simulink model "systema"  (R2017b)
settings: Solver=ode4  StartTime=0.0  StopTime=10  FixedStep=0.01  RelTol=1e-3  EnableMultiTasking=on
libraries: simulink x14
CloseFcn:
  | rtwprivate ssgencode ModelCloseRequest systema
settings Model: Creator=ece  LastModifiedBy=lenovo
settings DataIOCC: SaveFormat=Array  SignalLoggingName=sigsOut
settings OptimizationCC: OptimizeBlockIOStorage=off  BufferReuse=off  GlobalBufferReuse=off  ExpressionFolding=off  ExpressionDepthLimit=2147483647  LocalBlockOutputs=off  InitFltsAndDblsToZero=on  LifeSpan=inf
settings DebuggingCC: SaveWithParameterizedLinksMsg=none  UnderspecifiedInitializationDetection=Classic  MergeDetectMultiDrivingBlocksExec=none  SignalResolutionControl=TryResolveAllWithWarning  MultiTaskDSMMsg=warning  MultiTaskCondExecSysMsg=none  FcnCallInpInsideContextMsg=warning  AllowSymbolicDim=off  StateNameClashWarn=warning  SFUnexpectedBacktrackingDiag=warning  SFNoUnconditionalDefaultTransitionDiag=warning  SFExecutionAtInitializationDiag=none
settings HardwareCC: ProdBitPerPointer=32  ProdBitPerSizeT=32  ProdBitPerPtrDiffT=32  ProdLargestAtomicFloat=None  ProdIntDivRoundTo=Undefined  ProdEndianess=Unspecified  ProdWordSize=32  ProdHWDeviceType=32-bit Generic  TargetUnknown=on
settings ModelReferenceCC: PropagateSignalLabelsOutOfModel=off
settings CodeAppCC: StateflowObjectComments=on
settings GRTTargetCC: TargetFcnLib=ansi_tfl_tmw.mat  TargetLangStandard=C89/C90 (ANSI)  ModelReferenceCompliant=off  GeneratePreprocessorConditionals=Disable all  CombineOutputUpdateFcns=off  MatFileLogging=off  GRTInterface=on
settings ConfigComp: CovMetricSettings=dw  CovHtmlReporting=on  CovSaveCumulativeToWorkspaceVar=on  CovSaveSingleToWorkspaceVar=on  CovExternalEMLEnable=off

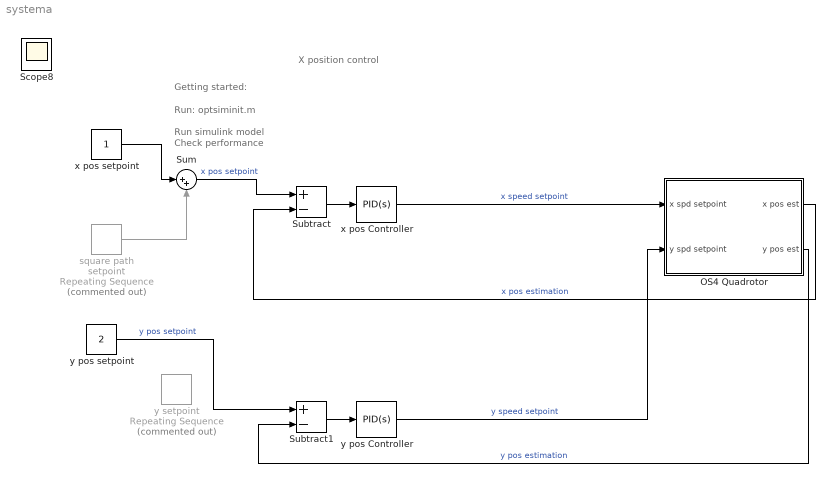
== system systema ==
  note: Check performance
  note: Run simulink model
  note: Run: optsiminit.m
  note: Getting started:
  note: X position control
  OS4 Quadrotor : Subsystem
  Subtract : Sum  Inputs=+-
  Subtract1 : Sum  Inputs=+-
  Sum : Sum  Inputs=|++
  square path setpoint : simulink/Sources/Repeating Sequence  Commented=on  rep_seq_t=[0 5 9.99 10 15 19.99 20 25]  rep_seq_y="[0 1 1       1 1 1 1 1]"
  x pos Controller : simulink/Continuous/PID Controller  Controller=PID  TimeDomain=Continuous-time  SampleTime=-1  IntegratorMethod=Forward Euler  FilterMethod=Forward Euler  Form=Parallel  UseFilter=on  ControllerParametersSource=internal  P=1.78976019221014  I=0.309124158830126  D=1.80752216558791  N=4.82597653544632  InitialConditionSource=internal  InitialConditionForIntegrator=0  InitialConditionForFilter=0  ExternalReset=none  LimitOutput=off  UpperSaturationLimit=inf  LowerSaturationLimit=-inf  LinearizeAsGain=off  AntiWindupMode=none  Kb=1  TrackingMode=off  Kt=1  PParamMin=[]  PParamMax=[]  IParamMin=[]  IParamMax=[]  DParamMin=[]  DParamMax=[]  NParamMin=[]  NParamMax=[]  KbParamMin=[]  KbParamMax=[]  KtParamMin=[]  KtParamMax=[]  POutMin=[]  POutMax=[]  IOutMin=[]  IOutMax=[]  DOutMin=[]  DOutMax=[]  NOutMin=[]  NOutMax=[]  KbOutMin=[]  KbOutMax=[]  KtOutMin=[]  KtOutMax=[]  IntegratorOutMin=[]  IntegratorOutMax=[]  FilterOutMin=[]  FilterOutMax=[]  SumOutMin=[]  SumOutMax=[]  SumI1OutMin=[]  SumI1OutMax=[]  SumI2OutMin=[]  SumI2OutMax=[]  SumI3OutMin=[]  SumI3OutMax=[]  SumDOutMin=[]  SumDOutMax=[]  SaturationOutMin=[]  SaturationOutMax=[]  IntegratorContinuousStateAttributes=''  IntegratorStateMustResolveToSignalObject=off  IntegratorRTWStateStorageClass=Auto  FilterContinuousStateAttributes=''  FilterStateMustResolveToSignalObject=off  FilterRTWStateStorageClass=Auto  DifferentiatorICPrevScaledInput=0  DifferentiatorOutMin=[]  DifferentiatorOutMax=[]  InitialConditionSetting=State (most efficient)  FilterDiffOutCoefMin=[]  FilterDiffOutCoefMax=[]  SumDenOutMin=[]  SumDenOutMax=[]  SumNumOutMin=[]  SumNumOutMax=[]  ReciprocalOutMin=[]  ReciprocalOutMax=[]  DivideOutMin=[]  DivideOutMax=[]  TunerSelectOption=Transfer Function Based (PID Tuner App)
  x pos setpoint : Constant
  y pos Controller : simulink/Continuous/PID Controller  Controller=PID  TimeDomain=Continuous-time  SampleTime=-1  IntegratorMethod=Forward Euler  FilterMethod=Forward Euler  Form=Parallel  UseFilter=on  ControllerParametersSource=internal  P=1  I=0.2  D=0  N=100  InitialConditionSource=internal  InitialConditionForIntegrator=0  InitialConditionForFilter=0  ExternalReset=none  LimitOutput=off  UpperSaturationLimit=inf  LowerSaturationLimit=-inf  LinearizeAsGain=off  AntiWindupMode=none  Kb=1  TrackingMode=off  Kt=1  PParamMin=[]  PParamMax=[]  IParamMin=[]  IParamMax=[]  DParamMin=[]  DParamMax=[]  NParamMin=[]  NParamMax=[]  KbParamMin=[]  KbParamMax=[]  KtParamMin=[]  KtParamMax=[]  POutMin=[]  POutMax=[]  IOutMin=[]  IOutMax=[]  DOutMin=[]  DOutMax=[]  NOutMin=[]  NOutMax=[]  KbOutMin=[]  KbOutMax=[]  KtOutMin=[]  KtOutMax=[]  IntegratorOutMin=[]  IntegratorOutMax=[]  FilterOutMin=[]  FilterOutMax=[]  SumOutMin=[]  SumOutMax=[]  SumI1OutMin=[]  SumI1OutMax=[]  SumI2OutMin=[]  SumI2OutMax=[]  SumI3OutMin=[]  SumI3OutMax=[]  SumDOutMin=[]  SumDOutMax=[]  SaturationOutMin=[]  SaturationOutMax=[]  IntegratorContinuousStateAttributes=''  IntegratorStateMustResolveToSignalObject=off  IntegratorRTWStateStorageClass=Auto  FilterContinuousStateAttributes=''  FilterStateMustResolveToSignalObject=off  FilterRTWStateStorageClass=Auto  DifferentiatorICPrevScaledInput=0  DifferentiatorOutMin=[]  DifferentiatorOutMax=[]  InitialConditionSetting=State (most efficient)  FilterDiffOutCoefMin=[]  FilterDiffOutCoefMax=[]  SumDenOutMin=[]  SumDenOutMax=[]  SumNumOutMin=[]  SumNumOutMax=[]  ReciprocalOutMin=[]  ReciprocalOutMax=[]  DivideOutMin=[]  DivideOutMax=[]  TunerSelectOption=Transfer Function Based (PID Tuner App)
  y pos setpoint : Constant  Value=2
  y setpoint : simulink/Sources/Repeating Sequence  Commented=on  rep_seq_t=[0 4.99 5 10 14.99 15 20 25]  rep_seq_y="[2 2   4 4 4 2 2 2]"
  Scope8 : Scope
  wires:
  Sum/1 -> Subtract/1  "x pos setpoint"
  Subtract/1 -> x pos Controller/1
  x pos Controller/1 -> OS4 Quadrotor/1(x spd setpoint)  "x speed setpoint"
  OS4 Quadrotor/1(x pos est) -> Subtract/2  "x pos estimation"
  square path setpoint/1 -> Sum/2
  x pos setpoint/1 -> Sum/1
  y pos setpoint/1 -> Subtract1/1  "y pos setpoint"
  Subtract1/1 -> y pos Controller/1
  y pos Controller/1 -> OS4 Quadrotor/2(y spd setpoint)  "y speed setpoint"
  OS4 Quadrotor/2(y pos est) -> Subtract1/2  "y pos estimation"

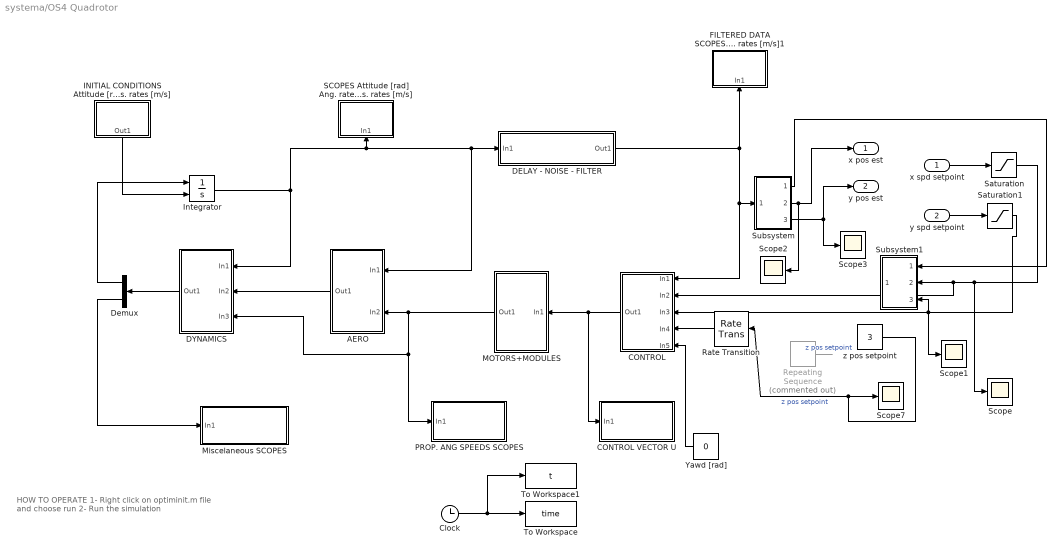
== system systema/OS4 Quadrotor ==
  note: HOW TO OPERATE
      | 1- Right click on optiminit.m file and choose run
      | 2- Run the simulation
  x spd setpoint : Inport
  y spd setpoint : Inport  Port=2
  AERO : Subsystem
  CONTROL : Subsystem
  CONTROL VECTOR U : Subsystem
  Clock : Clock
  DELAY - NOISE - FILTER : Subsystem
  DYNAMICS : Subsystem
  Demux : Demux  Outputs=2
  FILTERED DATA SCOPES Attitude [rad] Ang. rates [rad/sec] position [m] Pos. rates [m/s]1 : Subsystem
  "INITIAL CONDITIONS Attitude [rad] Ang. rates [rad/sec] position [m] Pos. rates [m/s] " : Subsystem
  Integrator : Integrator  InitialConditionSource=external
  MOTORS+MODULES : Subsystem
  Miscelaneous SCOPES : Subsystem
  PROP. ANG SPEEDS SCOPES : Subsystem
  Rate Transition : RateTransition
  Repeating Sequence : simulink/Sources/Repeating Sequence  Commented=on  rep_seq_t=[0 5 9.99 10 15 19.99 20 25]  rep_seq_y="[3 3 3       5 5 5 3 3]"
  SCOPES Attitude [rad] Ang. rates [rad/sec] position [m] Pos. rates [m/s] : Subsystem
  Saturation : Saturate  UpperLimit=20  LowerLimit=-20
  Saturation1 : Saturate  UpperLimit=20  LowerLimit=-20
  Scope{,1..3,7} (5 alike) : Scope
  Subsystem : Subsystem
  Subsystem1 : Subsystem
  To Workspace : ToWorkspace  VariableName=time  SampleTime=-1
  To Workspace1 : ToWorkspace  VariableName=t  SampleTime=-1
  Yawd [rad] : Constant  Value=0
  z pos setpoint : Constant  Value=3
  x pos est : Outport
  y pos est : Outport  Port=2
  wires:
  z pos setpoint/1 -> Scope7/1, Rate Transition/1  "z pos setpoint"
  Rate Transition/1 -> CONTROL/4(In4)
  y spd setpoint/1 -> Saturation1/1
  Saturation1/1 -> CONTROL/3(In3), Subsystem1/3(In3), Scope1/1
  Saturation/1 -> Scope/1, Subsystem1/2(In2), CONTROL/2(In2)
  x spd setpoint/1 -> Saturation/1
  Subsystem/1(Out2) -> Subsystem1/1(In1)
  Subsystem/2(Out3) -> x pos est/1, Scope2/1
  Subsystem/3(Out4) -> y pos est/1, Scope3/1
  DELAY - NOISE - FILTER/1(Out1) -> FILTERED DATA SCOPES Attitude [rad] Ang. rates [rad/sec] position [m] Pos. rates [m/s]1/1(In1), CONTROL/1(In1), Subsystem/1(In1)
  AERO/1(Out1) -> DYNAMICS/2(In2)
  MOTORS+MODULES/1(Out1) -> AERO/2(In2), DYNAMICS/3(In3), PROP. ANG SPEEDS SCOPES/1(In1)
  Yawd [rad]/1 -> CONTROL/5(In5)
  Demux/1 -> Integrator/1
  CONTROL/1(Out1) -> MOTORS+MODULES/1(In1), CONTROL VECTOR U/1(In1)
  Demux/2 -> Miscelaneous SCOPES/1(In1)
  DYNAMICS/1(Out1) -> Demux/1
  Clock/1 -> To Workspace/1, To Workspace1/1
  "INITIAL CONDITIONS Attitude [rad] Ang. rates [rad/sec] position [m] Pos. rates [m/s] "/1(Out1) -> Integrator/2
  Integrator/1 -> SCOPES Attitude [rad] Ang. rates [rad/sec] position [m] Pos. rates [m/s]/1(In1), DELAY - NOISE - FILTER/1(In1), AERO/1(In1), DYNAMICS/1(In1)
  Repeating Sequence/1 -> ?  "z pos setpoint"

== system systema/OS4 Quadrotor/AERO ==
  In1 : Inport
  In2 : Inport  Port=2
  AERO Attitude [rad] : MATLABFcn  MATLABFcn=aero  OutputDimensions=24
  Mux1 : Mux  Inputs=2
  Out1 : Outport
  wires:
  In1/1 -> Mux1/1
  In2/1 -> Mux1/2
  Mux1/1 -> AERO Attitude [rad]/1
  AERO Attitude [rad]/1 -> Out1/1

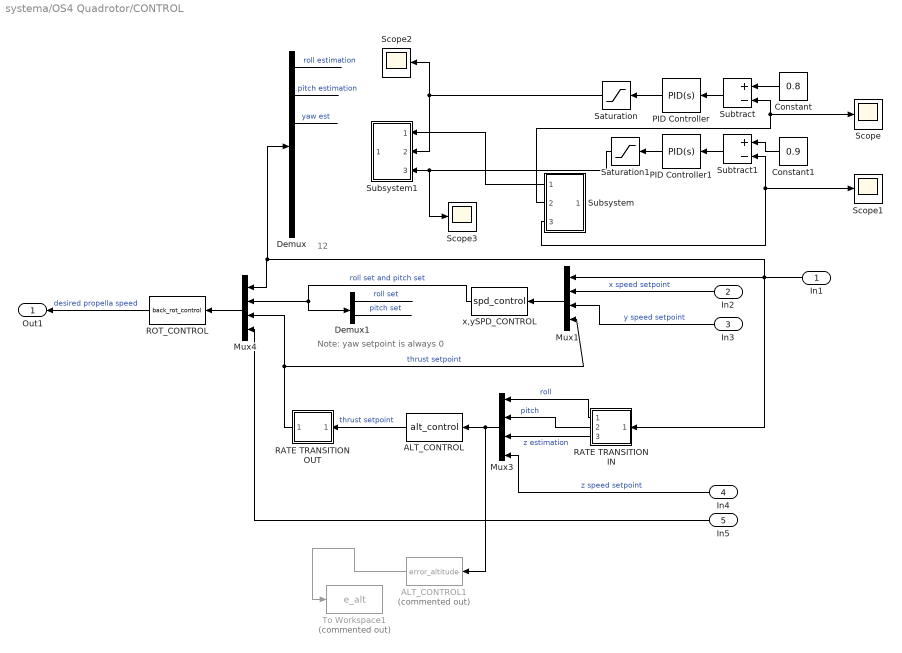
== system systema/OS4 Quadrotor/CONTROL ==
  note: Note: yaw setpoint is always 0
  note: 12
  In1 : Inport
  In2 : Inport  Port=2
  In3 : Inport  Port=3
  In4 : Inport  Port=4
  In5 : Inport  Port=5
  ALT_CONTROL : MATLABFcn  MATLABFcn=alt_control  OutputDimensions=1  SampleTime=0.05
  ALT_CONTROL1 : MATLABFcn  Commented=on  MATLABFcn=error_altitude  OutputDimensions=1  SampleTime=0.05
  Constant : Constant  Value=0.8
  Constant1 : Constant  Value=0.9
  Demux : Demux  Outputs=12
  Demux1 : Demux  Outputs=2
  Mux1 : Mux
  Mux3 : Mux
  Mux4 : Mux
  PID Controller : simulink/Continuous/PID Controller  Controller=PID  TimeDomain=Continuous-time  SampleTime=-1  IntegratorMethod=Forward Euler  FilterMethod=Forward Euler  Form=Parallel  UseFilter=on  ControllerParametersSource=internal  P=10  I=0.01  D=2  N=100  InitialConditionSource=internal  InitialConditionForIntegrator=0  InitialConditionForFilter=0  ExternalReset=none  LimitOutput=off  UpperSaturationLimit=inf  LowerSaturationLimit=-inf  LinearizeAsGain=off  AntiWindupMode=none  Kb=1  TrackingMode=off  Kt=1  PParamMin=[]  PParamMax=[]  IParamMin=[]  IParamMax=[]  DParamMin=[]  DParamMax=[]  NParamMin=[]  NParamMax=[]  KbParamMin=[]  KbParamMax=[]  KtParamMin=[]  KtParamMax=[]  POutMin=[]  POutMax=[]  IOutMin=[]  IOutMax=[]  DOutMin=[]  DOutMax=[]  NOutMin=[]  NOutMax=[]  KbOutMin=[]  KbOutMax=[]  KtOutMin=[]  KtOutMax=[]  IntegratorOutMin=[]  IntegratorOutMax=[]  FilterOutMin=[]  FilterOutMax=[]  SumOutMin=[]  SumOutMax=[]  SumI1OutMin=[]  SumI1OutMax=[]  SumI2OutMin=[]  SumI2OutMax=[]  SumI3OutMin=[]  SumI3OutMax=[]  SumDOutMin=[]  SumDOutMax=[]  SaturationOutMin=[]  SaturationOutMax=[]  IntegratorContinuousStateAttributes=''  IntegratorStateMustResolveToSignalObject=off  IntegratorRTWStateStorageClass=Auto  FilterContinuousStateAttributes=''  FilterStateMustResolveToSignalObject=off  FilterRTWStateStorageClass=Auto  DifferentiatorICPrevScaledInput=0  DifferentiatorOutMin=[]  DifferentiatorOutMax=[]  InitialConditionSetting=State (most efficient)  FilterDiffOutCoefMin=[]  FilterDiffOutCoefMax=[]  SumDenOutMin=[]  SumDenOutMax=[]  SumNumOutMin=[]  SumNumOutMax=[]  ReciprocalOutMin=[]  ReciprocalOutMax=[]  DivideOutMin=[]  DivideOutMax=[]  TunerSelectOption=Transfer Function Based (PID Tuner App)
  PID Controller1 : simulink/Continuous/PID Controller  Controller=PID  TimeDomain=Continuous-time  SampleTime=-1  IntegratorMethod=Forward Euler  FilterMethod=Forward Euler  Form=Parallel  UseFilter=on  ControllerParametersSource=internal  P=10  I=0.01  D=3  N=100  InitialConditionSource=internal  InitialConditionForIntegrator=0  InitialConditionForFilter=0  ExternalReset=none  LimitOutput=off  UpperSaturationLimit=inf  LowerSaturationLimit=-inf  LinearizeAsGain=off  AntiWindupMode=none  Kb=1  TrackingMode=off  Kt=1  PParamMin=[]  PParamMax=[]  IParamMin=[]  IParamMax=[]  DParamMin=[]  DParamMax=[]  NParamMin=[]  NParamMax=[]  KbParamMin=[]  KbParamMax=[]  KtParamMin=[]  KtParamMax=[]  POutMin=[]  POutMax=[]  IOutMin=[]  IOutMax=[]  DOutMin=[]  DOutMax=[]  NOutMin=[]  NOutMax=[]  KbOutMin=[]  KbOutMax=[]  KtOutMin=[]  KtOutMax=[]  IntegratorOutMin=[]  IntegratorOutMax=[]  FilterOutMin=[]  FilterOutMax=[]  SumOutMin=[]  SumOutMax=[]  SumI1OutMin=[]  SumI1OutMax=[]  SumI2OutMin=[]  SumI2OutMax=[]  SumI3OutMin=[]  SumI3OutMax=[]  SumDOutMin=[]  SumDOutMax=[]  SaturationOutMin=[]  SaturationOutMax=[]  IntegratorContinuousStateAttributes=''  IntegratorStateMustResolveToSignalObject=off  IntegratorRTWStateStorageClass=Auto  FilterContinuousStateAttributes=''  FilterStateMustResolveToSignalObject=off  FilterRTWStateStorageClass=Auto  DifferentiatorICPrevScaledInput=0  DifferentiatorOutMin=[]  DifferentiatorOutMax=[]  InitialConditionSetting=State (most efficient)  FilterDiffOutCoefMin=[]  FilterDiffOutCoefMax=[]  SumDenOutMin=[]  SumDenOutMax=[]  SumNumOutMin=[]  SumNumOutMax=[]  ReciprocalOutMin=[]  ReciprocalOutMax=[]  DivideOutMin=[]  DivideOutMax=[]  TunerSelectOption=Transfer Function Based (PID Tuner App)
  RATE TRANSITION IN : Subsystem
  RATE TRANSITION OUT : Subsystem
  ROT_CONTROL : MATLABFcn  MATLABFcn=back_rot_control  OutputDimensions=6
  Saturation : Saturate  UpperLimit=20  LowerLimit=-20
  Saturation1 : Saturate  UpperLimit=20  LowerLimit=-20
  Scope{,1..3} (4 alike) : Scope
  Subsystem : Subsystem
  Subsystem1 : Subsystem
  Subtract : Sum  Inputs=+-
  Subtract1 : Sum  Inputs=+-
  To Workspace1 : ToWorkspace  Commented=on  VariableName=e_alt  SampleTime=-1
  x,ySPD_CONTROL : MATLABFcn  MATLABFcn=spd_control  OutputDimensions=2
  Out1 : Outport
  wires:
  Mux1/1 -> x,ySPD_CONTROL/1
  ROT_CONTROL/1 -> Out1/1  "desired propella speed"
  In1/1 -> Mux1/1, RATE TRANSITION IN/1(In1), Demux/1, Mux4/1
  In2/1 -> Mux1/2  "x speed setpoint"
  x,ySPD_CONTROL/1 -> Demux1/1, Mux4/2  "roll set and pitch set"
  Mux4/1 -> ROT_CONTROL/1
  ALT_CONTROL/1 -> RATE TRANSITION OUT/1(In1)  "thrust setpoint"
  In5/1 -> Mux4/4
  RATE TRANSITION OUT/1(Out1) -> Mux4/3, Mux1/4  "thrust setpoint"
  Mux3/1 -> ALT_CONTROL/1, ALT_CONTROL1/1
  RATE TRANSITION IN/1(Out1) -> Mux3/1  "roll"
  RATE TRANSITION IN/2(Out2) -> Mux3/2  "pitch"
  RATE TRANSITION IN/3(Out3) -> Mux3/3  "z estimation"
  In4/1 -> Mux3/4  "z speed setpoint"
  In3/1 -> Mux1/3  "y speed setpoint"
  ALT_CONTROL1/1 -> To Workspace1/1
  Subtract/1 -> PID Controller/1
  Subtract1/1 -> PID Controller1/1
  Constant/1 -> Subtract/1
  Constant1/1 -> Subtract1/1
  PID Controller1/1 -> Saturation1/1
  PID Controller/1 -> Saturation/1
  Subsystem/1(Out2) -> Subsystem1/1(In1)
  Subsystem/2(Out3) -> Subtract/2, Scope/1
  Subsystem/3(Out4) -> Subtract1/2, Scope1/1
  Saturation/1 -> Subsystem1/2(In2), Scope2/1
  Saturation1/1 -> Subsystem1/3(In3), Scope3/1
  Demux/1 -> ?  "roll estimation"
  Demux/3 -> ?  "pitch estimation"
  Demux/5 -> ?  "yaw est"
  Demux1/1 -> ?  "roll set"
  Demux1/2 -> ?  "pitch set"

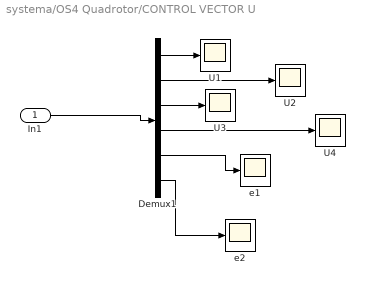
== system systema/OS4 Quadrotor/CONTROL VECTOR U ==
  In1 : Inport
  Demux1 : Demux  Outputs=6
  U{1..4} (4 alike) : Scope
  e1 : Scope
  e2 : Scope
  wires:
  In1/1 -> Demux1/1
  Demux1/4 -> U4/1
  Demux1/3 -> U3/1
  Demux1/2 -> U2/1
  Demux1/1 -> U1/1
  Demux1/5 -> e1/1
  Demux1/6 -> e2/1

== system systema/OS4 Quadrotor/DELAY - NOISE - FILTER ==
  In1 : Inport
  DELAYS : Subsystem
  LP FILTER : MATLABFcn  MATLABFcn=sam5_filter  OutputDimensions=12  OutputSignalType=real
  NOISY DATA SCOPES Attitude [rad] Ang. rates [rad/sec] position [m] Pos. rates [m/s]1 : Subsystem
  W. NORMAL NOISE1 : Subsystem
  Out1 : Outport
  wires:
  In1/1 -> DELAYS/1(In1)
  DELAYS/1(Out1) -> NOISY DATA SCOPES Attitude [rad] Ang. rates [rad/sec] position [m] Pos. rates [m/s]1/1(In1), LP FILTER/1
  LP FILTER/1 -> Out1/1

== system systema/OS4 Quadrotor/DYNAMICS ==
  In1 : Inport
  In2 : Inport  Port=2
  In3 : Inport  Port=3
  DYNAMICS : MATLABFcn  MATLABFcn=dinamica  OutputDimensions=18
  Mux1 : Mux  Inputs=3
  Out1 : Outport
  wires:
  DYNAMICS/1 -> Out1/1
  Mux1/1 -> DYNAMICS/1
  In2/1 -> Mux1/2
  In1/1 -> Mux1/1
  In3/1 -> Mux1/3

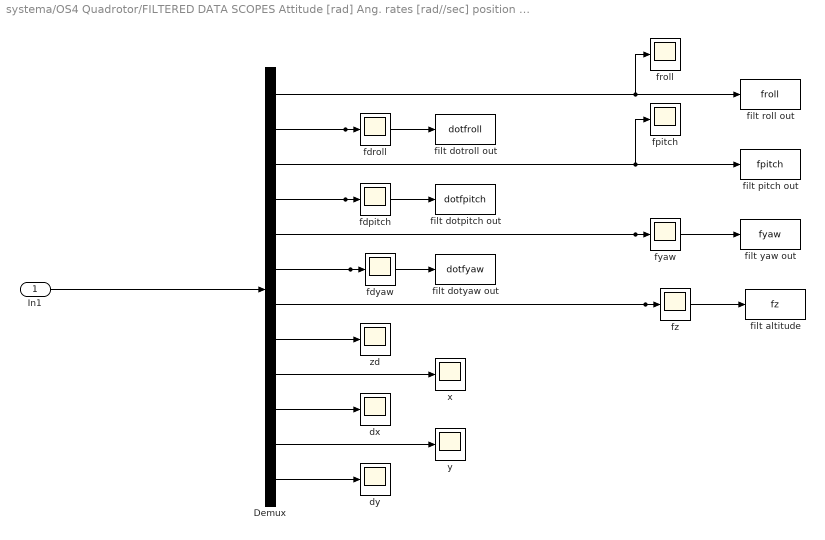
== system systema/OS4 Quadrotor/FILTERED DATA SCOPES Attitude [rad] Ang. rates [rad//sec] position [m] Pos. rates [m//s]1 ==
  In1 : Inport
  Demux : Demux  Outputs=12
  dx : Scope
  dy : Scope
  fdpitch : Scope
  fdroll : Scope
  fdyaw : Scope
  filt altitude : ToWorkspace  VariableName=fz  SampleTime=-1
  filt dotpitch out : ToWorkspace  VariableName=dotfpitch  SampleTime=-1
  filt dotroll out : ToWorkspace  VariableName=dotfroll  SampleTime=-1
  filt dotyaw out : ToWorkspace  VariableName=dotfyaw  SampleTime=-1
  filt pitch out : ToWorkspace  VariableName=fpitch  SampleTime=-1
  filt roll out : ToWorkspace  VariableName=froll  SampleTime=-1
  filt yaw out : ToWorkspace  VariableName=fyaw  SampleTime=-1
  fpitch : Scope
  froll : Scope
  fyaw : Scope
  fz : Scope
  x : Scope
  y : Scope
  zd : Scope
  wires:
  Demux/1 -> filt roll out/1, froll/1
  Demux/4 -> fdpitch/1, filt dotpitch out/1
  Demux/8 -> zd/1
  Demux/7 -> filt altitude/1, fz/1
  Demux/6 -> fdyaw/1, filt dotyaw out/1
  Demux/2 -> fdroll/1, filt dotroll out/1
  Demux/5 -> filt yaw out/1, fyaw/1
  Demux/3 -> filt pitch out/1, fpitch/1
  In1/1 -> Demux/1
  Demux/9 -> x/1
  Demux/10 -> dx/1
  Demux/11 -> y/1
  Demux/12 -> dy/1

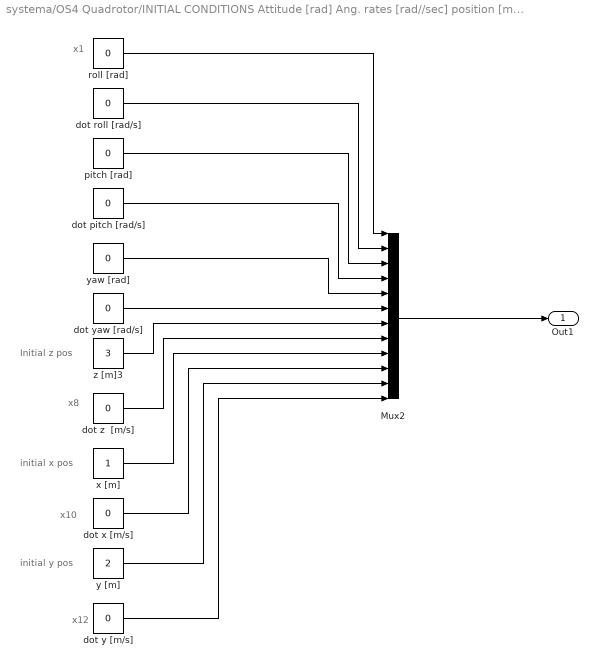
== system systema/OS4 Quadrotor/INITIAL CONDITIONS Attitude [rad] Ang. rates [rad//sec] position [m] Pos. rates [m//s]  ==
  note: initial y pos
  note: initial x pos
  note: Initial z pos
  note: x1
  note: x12
  note: x10
  note: x8
  Mux2 : Mux  Inputs=12
  dot pitch [rad/s] : Constant  Value=0
  dot roll [rad/s] : Constant  Value=0
  dot x [m/s] : Constant  Value=0
  dot y [m/s] : Constant  Value=0
  dot yaw [rad/s] : Constant  Value=0
  dot z  [m/s] : Constant  Value=0
  pitch [rad] : Constant  Value=0
  roll [rad] : Constant  Value=0
  x [m] : Constant
  y [m] : Constant  Value=2
  yaw [rad] : Constant  Value=0
  z [m]3 : Constant  Value=3
  Out1 : Outport
  wires:
  roll [rad]/1 -> Mux2/1
  dot roll [rad/s]/1 -> Mux2/2
  pitch [rad]/1 -> Mux2/3
  dot pitch [rad/s]/1 -> Mux2/4
  dot yaw [rad/s]/1 -> Mux2/6
  z [m]3/1 -> Mux2/7
  dot z  [m/s]/1 -> Mux2/8
  yaw [rad]/1 -> Mux2/5
  Mux2/1 -> Out1/1
  x [m]/1 -> Mux2/9
  dot x [m/s]/1 -> Mux2/10
  y [m]/1 -> Mux2/11
  dot y [m/s]/1 -> Mux2/12

== system systema/OS4 Quadrotor/MOTORS+MODULES ==
  In1 : Inport
  Bin2Om : MATLABFcn  MATLABFcn=bin2Om  OutputDimensions=4  OutputSignalType=real
  MOTOR DYNAMICS : Subsystem
  Saturation : Saturate  UpperLimit=125  LowerLimit=10
  U2bin : MATLABFcn  MATLABFcn=U2bin  OutputDimensions=4  OutputSignalType=real
  Out1 : Outport
  wires:
  Bin2Om/1 -> Out1/1
  MOTOR DYNAMICS/1(Out1) -> Bin2Om/1
  U2bin/1 -> Saturation/1
  In1/1 -> U2bin/1
  Saturation/1 -> MOTOR DYNAMICS/1(In1)

== system systema/OS4 Quadrotor/Miscelaneous SCOPES ==
  In1 : Inport  PortDimensions=6
  Demux : Demux  Outputs=6
  raa : Scope
  rgb : Scope
  rgp : Scope
  rhf : Scope
  rrm : Scope
  rrm1 : Scope
  wires:
  In1/1 -> Demux/1
  Demux/5 -> rrm/1
  Demux/4 -> rhf/1
  Demux/3 -> raa/1
  Demux/2 -> rgp/1
  Demux/1 -> rgb/1
  Demux/6 -> rrm1/1

== system systema/OS4 Quadrotor/PROP. ANG SPEEDS SCOPES ==
  In1 : Inport
  Demux1 : Demux
  omega{1..4} (4 alike) : Scope
  wires:
  Demux1/1 -> omega1/1
  Demux1/2 -> omega2/1
  Demux1/3 -> omega3/1
  Demux1/4 -> omega4/1
  In1/1 -> Demux1/1

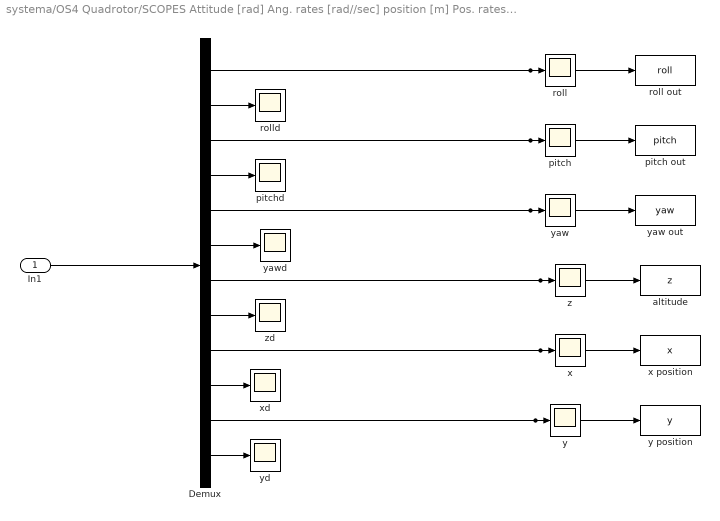
== system systema/OS4 Quadrotor/SCOPES Attitude [rad] Ang. rates [rad//sec] position [m] Pos. rates [m//s] ==
  In1 : Inport
  Demux : Demux  Outputs=12
  altitude : ToWorkspace  VariableName=z  SampleTime=-1
  pitch : Scope
  pitch out : ToWorkspace  VariableName=pitch  SampleTime=-1
  pitchd : Scope
  roll : Scope
  roll out : ToWorkspace  VariableName=roll  SampleTime=-1
  rolld : Scope
  x : Scope
  x position : ToWorkspace  VariableName=x  SampleTime=-1
  xd : Scope
  y : Scope
  y position : ToWorkspace  VariableName=y  SampleTime=-1
  yaw : Scope
  yaw out : ToWorkspace  VariableName=yaw  SampleTime=-1
  yawd : Scope
  yd : Scope
  z : Scope
  zd : Scope
  wires:
  In1/1 -> Demux/1
  Demux/3 -> pitch/1, pitch out/1
  Demux/5 -> yaw/1, yaw out/1
  Demux/2 -> rolld/1
  Demux/6 -> yawd/1
  Demux/7 -> z/1, altitude/1
  Demux/8 -> zd/1
  Demux/9 -> x/1, x position/1
  Demux/11 -> y/1, y position/1
  Demux/12 -> yd/1
  Demux/10 -> xd/1
  Demux/4 -> pitchd/1
  Demux/1 -> roll/1, roll out/1

== system systema/OS4 Quadrotor/Subsystem ==
  In1 : Inport
  Demux1 : Demux  Outputs=12
  Double click on this for demo.5 : Subsystem
      settings: OpenFcn=optsiminit
      mask Display: disp('optsiminit')
  Mux1 : Mux  Inputs=10
  Out2 : Outport
  Out3 : Outport  Port=2
  Out4 : Outport  Port=3
  wires:
  Demux1/1 -> Mux1/1
  Demux1/2 -> Mux1/2
  Demux1/3 -> Mux1/3
  Demux1/4 -> Mux1/4
  Demux1/5 -> Mux1/5
  Demux1/6 -> Mux1/6
  Demux1/7 -> Mux1/7
  Demux1/8 -> Mux1/8
  Demux1/10 -> Mux1/9
  Demux1/12 -> Mux1/10
  Mux1/1 -> Out2/1
  Demux1/9 -> Out3/1
  Demux1/11 -> Out4/1
  In1/1 -> Demux1/1

== system systema/OS4 Quadrotor/Subsystem1 ==
  In1 : Inport
  In2 : Inport  Port=2
  In3 : Inport  Port=3
  Demux1 : Demux  Outputs=10
  Mux1 : Mux  Inputs=12
  Out5 : Outport
  wires:
  In1/1 -> Demux1/1
  Demux1/1 -> Mux1/1
  Demux1/2 -> Mux1/2
  Demux1/3 -> Mux1/3
  Demux1/4 -> Mux1/4
  Demux1/5 -> Mux1/5
  Demux1/6 -> Mux1/6
  Demux1/7 -> Mux1/7
  Demux1/8 -> Mux1/8
  Demux1/10 -> Mux1/12
  Demux1/9 -> Mux1/10
  In2/1 -> Mux1/9
  In3/1 -> Mux1/11
  Mux1/1 -> Out5/1

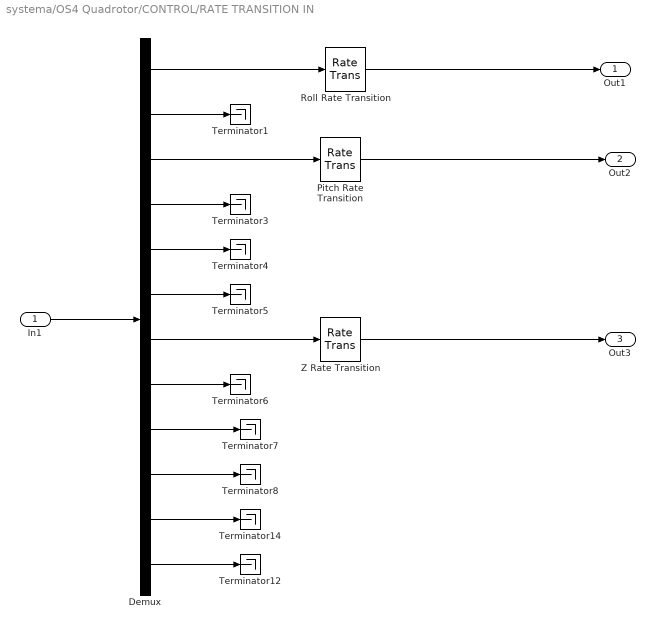
== system systema/OS4 Quadrotor/CONTROL/RATE TRANSITION IN ==
  In1 : Inport
  Demux : Demux  Outputs=12
  Pitch Rate Transition : RateTransition  Deterministic=off  OutPortSampleTime=50E-3
  Roll Rate Transition : RateTransition  Deterministic=off  OutPortSampleTime=50E-3
  Terminator{1,3..8,12,14} (9 alike) : Terminator
  Z Rate Transition : RateTransition  Deterministic=off  OutPortSampleTime=50E-3
  Out1 : Outport
  Out2 : Outport  Port=2
  Out3 : Outport  Port=3
  wires:
  Demux/7 -> Z Rate Transition/1
  In1/1 -> Demux/1
  Demux/1 -> Roll Rate Transition/1
  Demux/2 -> Terminator1/1
  Demux/3 -> Pitch Rate Transition/1
  Demux/4 -> Terminator3/1
  Demux/5 -> Terminator4/1
  Demux/6 -> Terminator5/1
  Demux/9 -> Terminator7/1
  Demux/10 -> Terminator8/1
  Demux/11 -> Terminator14/1
  Demux/12 -> Terminator12/1
  Demux/8 -> Terminator6/1
  Roll Rate Transition/1 -> Out1/1
  Pitch Rate Transition/1 -> Out2/1
  Z Rate Transition/1 -> Out3/1

== system systema/OS4 Quadrotor/CONTROL/RATE TRANSITION OUT ==
  In1 : Inport
  Rate Transition1 : RateTransition  Deterministic=off
  Out1 : Outport
  wires:
  In1/1 -> Rate Transition1/1
  Rate Transition1/1 -> Out1/1

== system systema/OS4 Quadrotor/CONTROL/Subsystem ==
  In1 : Inport
  Demux1 : Demux  Outputs=12
  Double click on this for demo.5 : Subsystem
      settings: OpenFcn=optsiminit
      mask Display: disp('optsiminit')
  Mux1 : Mux  Inputs=10
  Out2 : Outport
  Out3 : Outport  Port=2
  Out4 : Outport  Port=3
  wires:
  Demux1/1 -> Mux1/1
  Demux1/2 -> Mux1/2
  Demux1/3 -> Mux1/3
  Demux1/4 -> Mux1/4
  Demux1/5 -> Mux1/5
  Demux1/6 -> Mux1/6
  Demux1/7 -> Mux1/7
  Demux1/8 -> Mux1/8
  Demux1/10 -> Mux1/9
  Demux1/12 -> Mux1/10
  Mux1/1 -> Out2/1
  Demux1/9 -> Out3/1
  Demux1/11 -> Out4/1
  In1/1 -> Demux1/1

== system systema/OS4 Quadrotor/CONTROL/Subsystem1 ==
  In1 : Inport
  In2 : Inport  Port=2
  In3 : Inport  Port=3
  Demux1 : Demux  Outputs=10
  Mux1 : Mux  Inputs=12
  Out5 : Outport
  wires:
  In1/1 -> Demux1/1
  Demux1/1 -> Mux1/1
  Demux1/2 -> Mux1/2
  Demux1/3 -> Mux1/3
  Demux1/4 -> Mux1/4
  Demux1/5 -> Mux1/5
  Demux1/6 -> Mux1/6
  Demux1/7 -> Mux1/7
  Demux1/8 -> Mux1/8
  Demux1/10 -> Mux1/12
  Demux1/9 -> Mux1/10
  In2/1 -> Mux1/9
  In3/1 -> Mux1/11
  Mux1/1 -> Out5/1

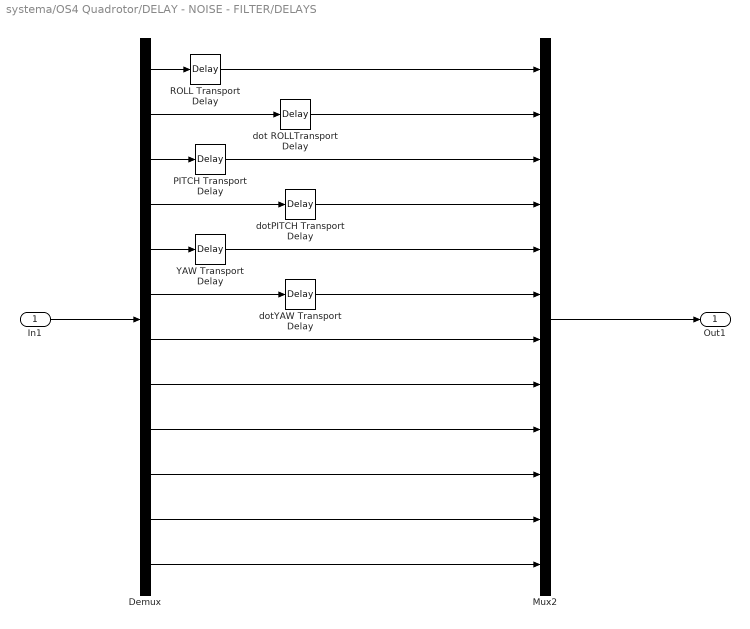
== system systema/OS4 Quadrotor/DELAY - NOISE - FILTER/DELAYS ==
  In1 : Inport
  Demux : Demux  Outputs=12
  Mux2 : Mux  Inputs=12
  PITCH Transport Delay : TransportDelay  DelayTime=8E-3
  ROLL Transport Delay : TransportDelay  DelayTime=8E-3
  YAW Transport Delay : TransportDelay  DelayTime=8E-3
  dot ROLLTransport Delay : TransportDelay  DelayTime=4.5E-3
  dotPITCH Transport Delay : TransportDelay  DelayTime=4.5E-3
  dotYAW Transport Delay : TransportDelay  DelayTime=4.5E-3
  Out1 : Outport
  wires:
  dot ROLLTransport Delay/1 -> Mux2/2
  Demux/12 -> Mux2/12
  Demux/11 -> Mux2/11
  Demux/10 -> Mux2/10
  Demux/9 -> Mux2/9
  Demux/8 -> Mux2/8
  Demux/7 -> Mux2/7
  dotYAW Transport Delay/1 -> Mux2/6
  Demux/6 -> dotYAW Transport Delay/1
  YAW Transport Delay/1 -> Mux2/5
  Demux/5 -> YAW Transport Delay/1
  dotPITCH Transport Delay/1 -> Mux2/4
  Demux/4 -> dotPITCH Transport Delay/1
  PITCH Transport Delay/1 -> Mux2/3
  Demux/3 -> PITCH Transport Delay/1
  Demux/2 -> dot ROLLTransport Delay/1
  ROLL Transport Delay/1 -> Mux2/1
  Demux/1 -> ROLL Transport Delay/1
  In1/1 -> Demux/1
  Mux2/1 -> Out1/1

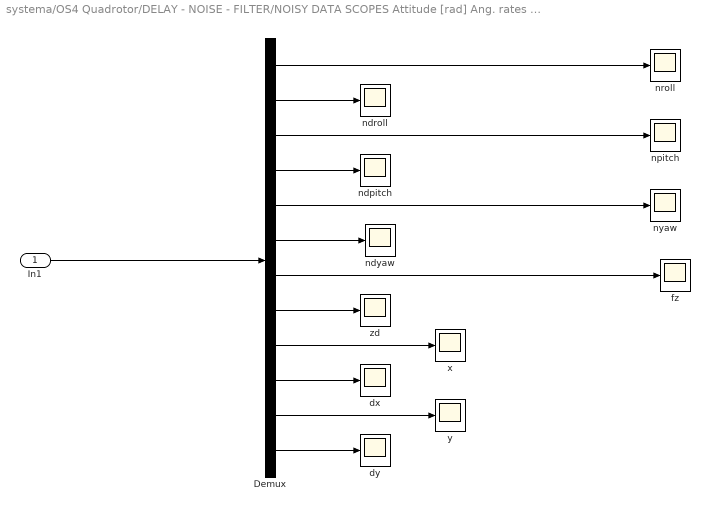
== system systema/OS4 Quadrotor/DELAY - NOISE - FILTER/NOISY DATA SCOPES Attitude [rad] Ang. rates [rad//sec] position [m] Pos. rates [m//s]1 ==
  In1 : Inport
  Demux : Demux  Outputs=12
  dx : Scope
  dy : Scope
  fz : Scope
  ndpitch : Scope
  ndroll : Scope
  ndyaw : Scope
  npitch : Scope
  nroll : Scope
  nyaw : Scope
  x : Scope
  y : Scope
  zd : Scope
  wires:
  Demux/1 -> nroll/1
  Demux/4 -> ndpitch/1
  Demux/8 -> zd/1
  Demux/7 -> fz/1
  Demux/6 -> ndyaw/1
  Demux/2 -> ndroll/1
  Demux/5 -> nyaw/1
  Demux/3 -> npitch/1
  In1/1 -> Demux/1
  Demux/9 -> x/1
  Demux/10 -> dx/1
  Demux/11 -> y/1
  Demux/12 -> dy/1

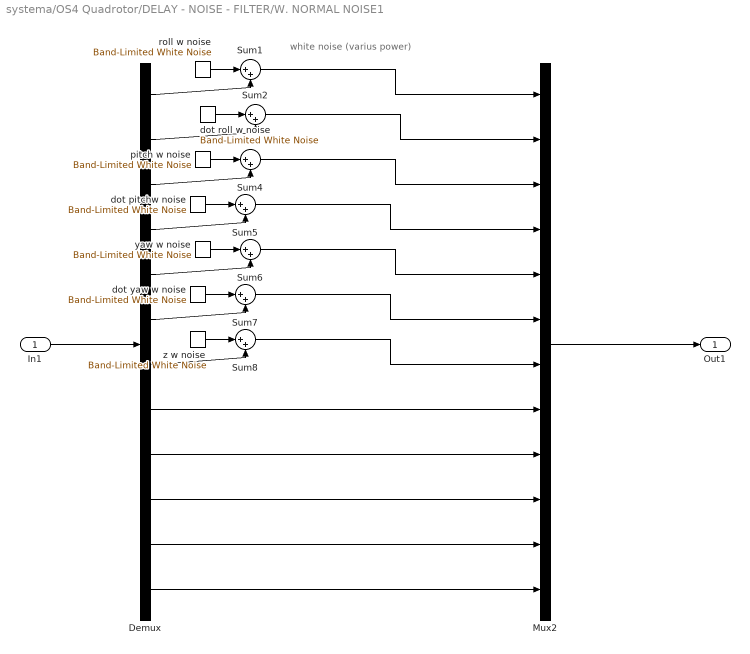
== system systema/OS4 Quadrotor/DELAY - NOISE - FILTER/W. NORMAL NOISE1 ==
  note: white noise (varius power)
  In1 : Inport
  Demux : Demux  Outputs=12
  Mux2 : Mux  Inputs=12
  Sum{1..2,4..8} (7 alike) : Sum  Inputs=|++  SaturateOnIntegerOverflow=on
  dot pitchw noise : simulink/Sources/Band-Limited White Noise  Cov=[0.0001]  Ts=0.01  seed=[23341]
  dot roll w noise : simulink/Sources/Band-Limited White Noise  Cov=[0.0001]  Ts=0.01  seed=[23341]
  dot yaw w noise : simulink/Sources/Band-Limited White Noise  Cov=[0.0001]  Ts=0.01  seed=[23341]
  pitch w noise : simulink/Sources/Band-Limited White Noise  Cov=[0.00001]  Ts=0.01  seed=[23341]
  roll w noise : simulink/Sources/Band-Limited White Noise  Cov=[0.00001]  Ts=0.01  seed=[24431]
  yaw w noise : simulink/Sources/Band-Limited White Noise  Cov=[0.00001]  Ts=0.01  seed=[23341]
  z w noise : simulink/Sources/Band-Limited White Noise  Cov=[0.00001]  Ts=0.01  seed=[23341]
  Out1 : Outport
  wires:
  Demux/8 -> Mux2/8
  Demux/12 -> Mux2/12
  Demux/11 -> Mux2/11
  Demux/10 -> Mux2/10
  Demux/9 -> Mux2/9
  Sum8/1 -> Mux2/7
  z w noise/1 -> Sum8/1
  Demux/7 -> Sum8/2
  Sum7/1 -> Mux2/6
  dot yaw w noise/1 -> Sum7/1
  Demux/6 -> Sum7/2
  Sum6/1 -> Mux2/5
  yaw w noise/1 -> Sum6/1
  Demux/5 -> Sum6/2
  Sum5/1 -> Mux2/4
  dot pitchw noise/1 -> Sum5/1
  Demux/4 -> Sum5/2
  Sum4/1 -> Mux2/3
  pitch w noise/1 -> Sum4/1
  Demux/3 -> Sum4/2
  Sum2/1 -> Mux2/2
  dot roll w noise/1 -> Sum2/1
  Demux/2 -> Sum2/2
  Sum1/1 -> Mux2/1
  roll w noise/1 -> Sum1/1
  Mux2/1 -> Out1/1
  In1/1 -> Demux/1
  Demux/1 -> Sum1/2

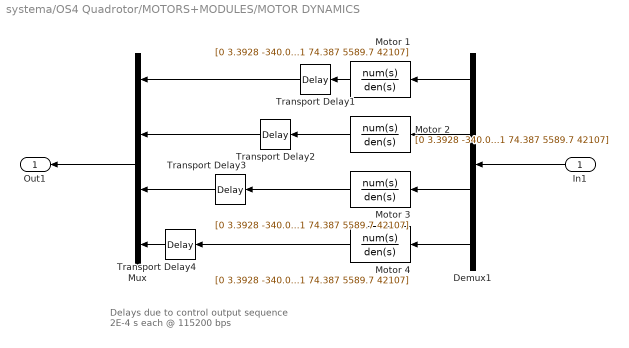
== system systema/OS4 Quadrotor/MOTORS+MODULES/MOTOR DYNAMICS ==
  note: Delays due to control output sequence
      | 2E-4 s each @ 115200 bps
  In1 : Inport
  Demux1 : Demux
  Motor {1..4} (4 alike) : TransferFcn  Numerator=[0 3.3928 -340.09 39451]  Denominator=[1 74.387 5589.7 42107]
  Mux : Mux
  Transport Delay1 : TransportDelay  DelayTime=2E-4
  Transport Delay2 : TransportDelay  DelayTime=4E-4
  Transport Delay3 : TransportDelay  DelayTime=6E-4
  Transport Delay4 : TransportDelay  DelayTime=8E-4
  Out1 : Outport
  wires:
  In1/1 -> Demux1/1
  Demux1/1 -> Motor 1/1
  Demux1/2 -> Motor 2/1
  Demux1/3 -> Motor 3/1
  Demux1/4 -> Motor 4/1
  Motor 1/1 -> Transport Delay1/1
  Motor 2/1 -> Transport Delay2/1
  Motor 3/1 -> Transport Delay3/1
  Motor 4/1 -> Transport Delay4/1
  Mux/1 -> Out1/1
  Transport Delay2/1 -> Mux/2
  Transport Delay3/1 -> Mux/3
  Transport Delay4/1 -> Mux/4
  Transport Delay1/1 -> Mux/1

== system systema/OS4 Quadrotor/Subsystem/Double click on this for demo.5 ==

== system systema/OS4 Quadrotor/CONTROL/Subsystem/Double click on this for demo.5 ==
